simulink model "Bldc_running"  (R2025a)
settings: Solver=VariableStepAuto  StartTime=0.0  StopTime=1  RelTol=1e-3
libraries: spsIGBTDiodeLib x6, spsDCVoltageSourceLib x1, spsGroundLib x1, spsVoltageMeasurementLib x1, spsPermanentMagnetSynchronousMachineLib x1, spsThreePhaseVIMeasurementLib x1, sps_lib x1
settings Model: Creator=mugun  LastModifiedBy=mugun

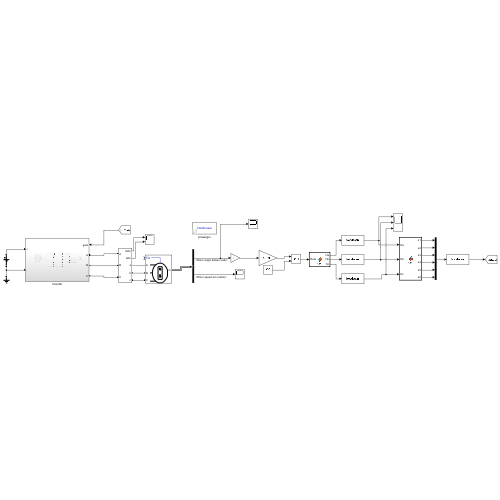
[thumbnail: Simulink's stored preview of the top-level diagram]
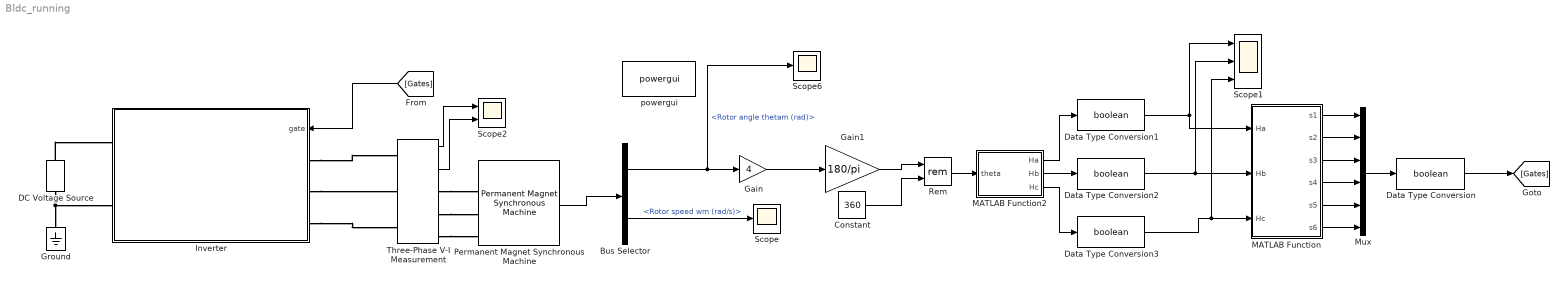
== system Bldc_running ==
  Bus Selector : BusSelector  OutputSignals=Rotor angle thetam (rad),Rotor speed wm (rad/s)
  Constant : Constant  Value=360
  DC Voltage Source : spsDCVoltageSourceLib/DC Voltage Source  Amplitude=100  Measurements=None
  Data Type Conversion{,1..3} (4 alike) : DataTypeConversion  OutDataTypeStr=boolean  SaturateOnIntegerOverflow=off  RndMeth=Floor
  Gain : Gain  Gain=4
  Gain1 : Gain  Gain=180/pi
  Ground : spsGroundLib/Ground  LConnTagsString=a
  Inverter : Subsystem
      settings: PortSchema="{\"entries\":[{\"content\":{\"sides\":[{\"content\":{\"connectorIds\":[\"LConn1\",\"LConn2\"]},\"type\":\"ConnectorPlacement.EquallySpacedRectSide\",\"uuid\":\"18219423-8b1f-43e6-a43a-6c4945a1488d\"},{\"content\":{\"connectorIds\":[\"In1\",\"RConn1\",\"RConn2\",\"RConn3\"],\"side\":\"RIGHT\"},\"type\":\"ConnectorPlacement.EquallySpacedRectSide\",\"uuid\":\"d63a9969-6ec8-4e38-b2d2-b97f72faf8f7\"},{\"content\":{\"side\":\"TOP\"},\"type\":\"ConnectorPlacement.EquallySpacedRectSide\",\"uuid\":\"5719017d-d8ee-42b1-98fe-ac6ef4c4d1f0\"}]},\"type\":\"ConnectorPlacement.EquallySpacedConnector\",\"uuid\":\"d6ba9602-361d-4528-9af6-3ebb689ccd27\"}],\"packageUris\":[\"http://schema.mathworks.com/mf0/Connector/R2020b\"],\"version\":\"1.0\"}"
  MATLAB Function : MATLAB Function  TreatAsAtomicUnit=on
  MATLAB Function2 : MATLAB Function  TreatAsAtomicUnit=on
  Mux : Mux  Inputs=6
  Permanent Magnet Synchronous Machine : spsPermanentMagnetSynchronousMachineLib/Permanent Magnet Synchronous Machine  NbPhases=3  FluxDistribution=Trapezoidal  RotorType=Round  MechanicalLoad=Torque Tm  PresetModel=No  ShowDetailedParameters=on  MeasurementBus=off  Resistance=0.0485  Inductance=8.5e-3  dqInductances=[8.5e-3,8.5e-3]  La=0.000395  MachineConstant=Flux linkage established by magnets (V.s)  Flux=0.1194  VoltageCst=100.0283  TorqueCst=0.9552  Flat=120  Mechanical=[0.0027 0.0004924 4 0]  PolePairs=4  InitialConditions=[0,0, 0,0]  InitialConditions5ph=[0 0 0 0 0 0]  RefAngle=90 degrees behind phase A axis (modified Park)  IterativeDiscreteModel=Trapezoidal non iterative  TsBlock=-1  TsPowergui=0
  Rem : Math  Operator=rem
  Scope : Scope
      settings: ActiveDisplayYMinimum=-14.680286950216473  ActiveDisplayYMaximum=159.25676169885932
  Scope1 : Scope  NumInputPorts=3
      settings: ActiveDisplayYMinimum=-0.12499999999999997  ActiveDisplayYMaximum=1.125
  Scope2 : Scope  NumInputPorts=2
      settings: ActiveDisplayYMinimum=39.999999999999993  ActiveDisplayYMaximum=59.999999999999993  DataLoggingVariableName=ScopeData2
  Scope6 : Scope
      settings: ActiveDisplayYMinimum=-1  ActiveDisplayYMaximum=1  DataLoggingVariableName=ScopeData6
  Three-Phase V-I Measurement : spsThreePhaseVIMeasurementLib/Three-Phase V-I Measurement  VoltageMeasurement=phase-to-ground  SetLabelV=off  LabelV=Vabc  Vpu=off  VpuLL=off  CurrentMeasurement=yes  SetLabelI=off  LabelI=Iabc  Ipu=off  Pbase=100e6  Vbase=500e3  OutputType=Complex  PhasorSimulation=off  PSBequivalent=0
  powergui : sps_lib/powergui  Priority=1  SimulationMode=Continuous  SampleTime=50e-6  frequency=60  Iterations=50  frequencyindice=0  Pbase=100e6  ErrMax=1e-4  UnitsV=kV  UnitsW=MW  buscounter=0  FunctionMessages=off  echomessages=off  EnableUseOfTLC=off  CurrentSourceSwitches=off  DisableSnubberDevices=off  DisableRonSwitches=off  DisableVfSwitches=off  DisplayEquations=off  AutomaticDiscreteSolvers=off  SolverType=Tustin/Backward Euler (TBE)  Interpol=off  ExternalGateDelay=off  methode=off  Ts=100  x0status=blocks  SPID=on  SwTol=0  HookPort=off  NonlinearTolerance=1e-4  nMaxIteration=100  ContinueOnMaxIteration=off  RestoreLinks=warning  ResistiveCurrentMeasurement=off  Frange=[0:2:500]  Ylog=off  Xlog=on  ShowGrid=off  save=off  variable=ZData  structure=0  ZoomFFT=off  StartTime=0.0  cycles=1  DisplayStyle=1  fundamental=60  FreqAxis=off  MaxFrequency=1000  frequencyindicesteady=1  RmsSteady=1  display=off
  wires:
  Permanent Magnet Synchronous Machine/1 -> Bus Selector/1
  Bus Selector/1 -> Scope6/1, Gain/1  "<Rotor angle thetam (rad)>"
  Gain/1 -> Gain1/1
  Gain1/1 -> Rem/1
  Constant/1 -> Rem/2
  Rem/1 -> MATLAB Function2/1(theta)
  Bus Selector/2 -> Scope/1  "<Rotor speed wm (rad/s)>"
  MATLAB Function/1(s1) -> Mux/1
  MATLAB Function/2(s2) -> Mux/2
  MATLAB Function/3(s3) -> Mux/3
  MATLAB Function/4(s4) -> Mux/4
  MATLAB Function/5(s5) -> Mux/5
  MATLAB Function/6(s6) -> Mux/6
  Three-Phase V-I Measurement/1 -> Scope2/1
  Three-Phase V-I Measurement/2 -> Scope2/2
  Mux/1 -> Data Type Conversion/1
  Data Type Conversion/1 -> [Gates]
  [Gates] -> Inverter/1(gate)
  MATLAB Function2/1(Ha) -> Data Type Conversion1/1
  MATLAB Function2/2(Hb) -> Data Type Conversion2/1
  MATLAB Function2/3(Hc) -> Data Type Conversion3/1
  Data Type Conversion1/1 -> MATLAB Function/1(Ha), Scope1/1
  Data Type Conversion2/1 -> Scope1/2, MATLAB Function/2(Hb)
  Data Type Conversion3/1 -> Scope1/3, MATLAB Function/3(Hc)
  connections:
  DC Voltage Source/LConn1 -- Ground/LConn1 -- Inverter/LConn2
  Three-Phase V-I Measurement/RConn1 -- Permanent Magnet Synchronous Machine/LConn1
  Three-Phase V-I Measurement/RConn2 -- Permanent Magnet Synchronous Machine/LConn2
  Three-Phase V-I Measurement/RConn3 -- Permanent Magnet Synchronous Machine/LConn3
  Inverter/RConn1 -- Three-Phase V-I Measurement/LConn1
  Inverter/RConn2 -- Three-Phase V-I Measurement/LConn2
  Inverter/RConn3 -- Three-Phase V-I Measurement/LConn3
  DC Voltage Source/RConn1 -- Inverter/LConn1

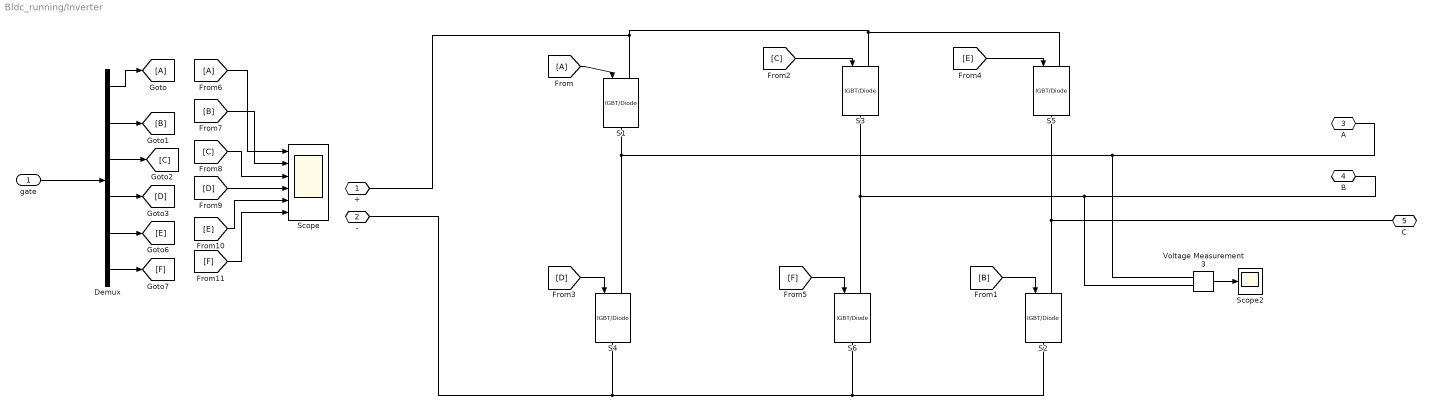
== system Bldc_running/Inverter ==
  gate : Inport
  Demux : Demux  Outputs=6
  From : From
  From6 : From
  Goto : Goto
  S{1..6} (6 alike) : spsIGBTDiodeLib/IGBT//Diode  Ron=1e-3  Rs=1e5  Cs=inf  Measurements=off
  Scope : Scope  NumInputPorts=6
      settings: ActiveDisplayYMinimum=-0.12499999999999997  ActiveDisplayYMaximum=1.125
  Scope2 : Scope
      settings: ActiveDisplayYMinimum=-125.04211749866226  ActiveDisplayYMaximum=125.01656195858735  DataLoggingVariableName=ScopeData3
  Voltage Measurement3 : spsVoltageMeasurementLib/Voltage Measurement  PhasorSimulation=off  OutputType=Complex  PSBequivalent=0
  + : PMIOPort  Side=Left
  - : PMIOPort  Port=2  Side=Left
  A : PMIOPort  Port=3  Side=Right
  B : PMIOPort  Port=4  Side=Right
  C : PMIOPort  Port=5  Side=Right
  wires:
  [F] -> Scope/6
  From/1 -> S1/1
  [D] -> Scope/4
  [F] -> S6/1
  [C] -> S3/1
  Demux/2 -> [B]
  Demux/1 -> Goto/1
  [D] -> S4/1
  Demux/3 -> [C]
  From6/1 -> Scope/1
  [B] -> Scope/2
  [C] -> Scope/3
  gate/1 -> Demux/1
  [B] -> S2/1
  [E] -> S5/1
  Demux/4 -> [D]
  Demux/5 -> [E]
  [E] -> Scope/5
  Voltage Measurement3/1 -> Scope2/1
  Demux/6 -> [F]
  connections:
  S2/RConn1 -- S6/RConn1 -- -/RConn1 -- S4/RConn1
  Voltage Measurement3/LConn2 -- S3/RConn1 -- S6/LConn1 -- B/RConn1
  S5/RConn1 -- S2/LConn1 -- C/RConn1
  S4/LConn1 -- S1/RConn1 -- A/RConn1 -- Voltage Measurement3/LConn1
  S5/LConn1 -- S3/LConn1 -- S1/LConn1 -- +/RConn1

== matlab function Bldc_running/MATLAB Function ==
  data: Ha input; s1 output; Hb input; Hc input; s2 output; s3 output; s4 output; s5 output; s6 output
function [s1,s2,s3,s4,s5,s6] = fcn(Ha,Hb,Hc)

if (Ha==1 && Hb==0 && Hc==1)
    s1=1;s2=1;s3=0;s4=0;s5=0;s6=0;

elseif (Ha==1 && Hb==0 && Hc==0)
    s1=0;s2=1;s3=1;s4=0;s5=0;s6=0;

elseif (Ha==1 && Hb==1 && Hc==0)
    s1=0;s2=0;s3=1;s4=1;s5=0;s6=0;

elseif (Ha==0 && Hb==1 && Hc==0)
    s1=0;s2=0;s3=0;s4=1;s5=1;s6=0;

elseif (Ha==0 && Hb==1 && Hc==1)
    s1=0;s2=0;s3=0;s4=0;s5=1;s6=1;

elseif (Ha==0 && Hb==0 && Hc==1)
    s1=1;s2=0;s3=0;s4=0;s5=0;s6=1;

else 
    s1=0;s2=0;s3=0;s4=0;s5=0;s6=0;

end

== matlab function Bldc_running/MATLAB Function2 ==
  data: theta input; Ha output; Hb output; Hc output
function [Ha,Hb,Hc] = fcn(theta)

if (theta>330 && theta<=360) || (theta>=0 && theta<=30)
    Ha=1;
    Hb=0;
    Hc=1;

elseif (theta>30 && theta<=90)
    Ha=1;
    Hb=0;
    Hc=0;
elseif (theta>90 && theta<=150)
    Ha=1;
    Hb=1;
    Hc=0;
elseif (theta>150 && theta<=210)
    Ha=0;
    Hb=1;
    Hc=0;
elseif (theta>210 && theta<=270)
    Ha=0;
    Hb=1;
    Hc=1;
elseif (theta>270 && theta<=330)
    Ha=0;
    Hb=0;
    Hc=1;
else
    Ha=0;
    Hb=0;
    Hc=0;
end
